simulink model "Pose_integration_R_L"  (R2016b)
settings: Solver=FixedStepDiscrete  StartTime=0.0  StopTime=60  FixedStep=0.02  RelTol=1e-3  EnableMultiTasking=on
InitFcn:
  | load('Pose_integration_R_L.mat')
StopFcn:
  | I = imread('Enviroment.png');
  | x = [0 35.9];
  | y=[23.31 0];
  | image(I,'XData',x,'YData',y);
  | axis xy;
  | hold on
  | plot (X.Data, Y.Data,'b');
  | plot (X1.Data, Y1.Data,'r');
undefined symbols (not defined in the file or in its folder): DiscIntNeverNeededParam, Ts
settings Model: Creator=antonio  LastModifiedBy=Antonio
settings DataIOCC: LimitDataPoints=on  SaveFormat=Array
settings OptimizationCC: LifeSpan=inf
settings DebuggingCC: UnderspecifiedInitializationDetection=Classic  MergeDetectMultiDrivingBlocksExec=none  SolverPrmCheckMsg=warning  StateNameClashWarn=warning  SFUnexpectedBacktrackingDiag=warning  SFNoUnconditionalDefaultTransitionDiag=warning  SFExecutionAtInitializationDiag=none
settings HardwareCC: ProdBitPerPointer=32  ProdBitPerSizeT=32  ProdBitPerPtrDiffT=32  ProdLargestAtomicFloat=None  ProdIntDivRoundTo=Undefined  ProdEndianess=Unspecified  ProdWordSize=32  ProdHWDeviceType=32-bit Generic
settings ModelReferenceCC: PropagateSignalLabelsOutOfModel=off
settings GRTTargetCC: TargetLangStandard=C89/C90 (ANSI)  GeneratePreprocessorConditionals=Disable all
settings ConfigComp: CovMetricSettings=dw  CovHtmlReporting=on  CovSaveCumulativeToWorkspaceVar=on  CovSaveSingleToWorkspaceVar=on  CovExternalEMLEnable=off

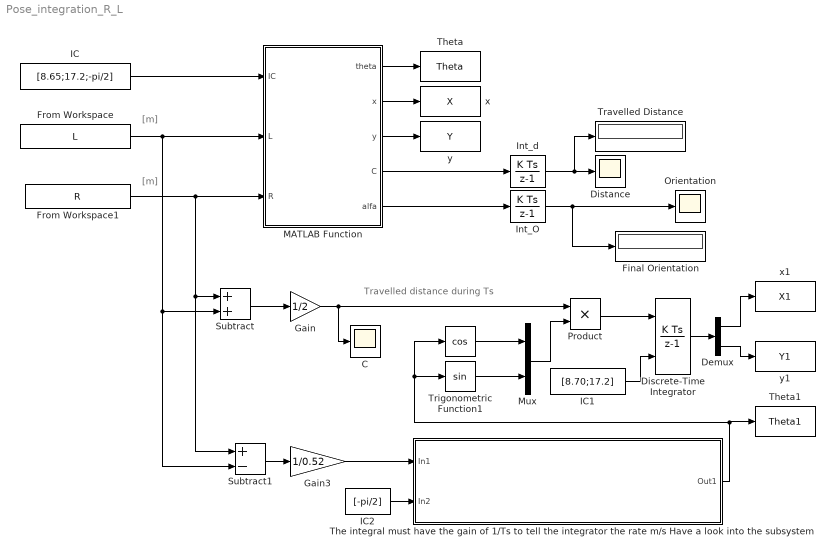
== system Pose_integration_R_L ==
  note: Travelled distance during Ts
  note: [m]
  note: [m]
  " " : Trigonometry  Operator=cos
  C : Scope
  Demux : Demux  Outputs=2
  Discrete-Time Integrator : DiscreteIntegrator  gainval=1/Ts  InitialConditionSource=external  InitialConditionSetting=State (most efficient)  SampleTime=Ts  ICPrevOutput=DiscIntNeverNeededParam  ICPrevScaledInput=DiscIntNeverNeededParam
  Distance : Scope
  Final Orientation : Display
  From Workspace : FromWorkspace  VariableName=L  SampleTime=0
  From Workspace1 : FromWorkspace  VariableName=R  SampleTime=0
  Gain : Gain  Gain=1/2
  Gain3 : Gain  Gain=1/0.52
  IC : Constant  Value=[8.65;17.2;-pi/2]
  IC1 : Constant  Value=[8.70;17.2]
  IC2 : Constant  Value=[-pi/2]
  Int_O : DiscreteIntegrator  gainval=1/Ts  InitialCondition=-pi/2  InitialConditionSetting=State (most efficient)  SampleTime=Ts  ICPrevOutput=DiscIntNeverNeededParam  ICPrevScaledInput=DiscIntNeverNeededParam
  Int_d : DiscreteIntegrator  gainval=1/Ts  InitialConditionSetting=State (most efficient)  SampleTime=Ts  ICPrevOutput=DiscIntNeverNeededParam  ICPrevScaledInput=DiscIntNeverNeededParam
  MATLAB Function : MATLAB Function  TreatAsAtomicUnit=on
  Mux : Mux  Inputs=2
  Orientation : Scope
  Product : Product
  Subtract : Sum
  Subtract1 : Sum  Inputs=+-
  The integral must have the gain of 1/Ts to tell the integrator the rate m/s Have a look into the subsystem : Subsystem
      mask Display: image('Integral.jpg');
  Theta : ToWorkspace  VariableName=Theta  SaveFormat=Timeseries  SampleTime=-1
  Theta1 : ToWorkspace  VariableName=Theta1  SaveFormat=Timeseries  SampleTime=-1
  Travelled Distance : Display
  Trigonometric Function1 : Trigonometry
  x : ToWorkspace  VariableName=X  SaveFormat=Timeseries  SampleTime=-1
  x1 : ToWorkspace  VariableName=X1  SaveFormat=Timeseries  SampleTime=-1
  y : ToWorkspace  VariableName=Y  SaveFormat=Timeseries  SampleTime=-1
  y1 : ToWorkspace  VariableName=Y1  SaveFormat=Timeseries  SampleTime=-1
  wires:
  IC/1 -> MATLAB Function/1(IC)
  MATLAB Function/1(theta) -> Theta/1
  MATLAB Function/3(y) -> y/1
  MATLAB Function/2(x) -> x/1
  From Workspace1/1 -> Subtract1/1, Subtract/1, MATLAB Function/3(R)
  From Workspace/1 -> MATLAB Function/2(L), Subtract1/2, Subtract/2
  Subtract/1 -> Gain/1
  Gain/1 -> C/1, Product/1
  Trigonometric Function1/1 -> Mux/2
  " "/1 -> Mux/1
  Mux/1 -> Product/2
  Subtract1/1 -> Gain3/1
  Product/1 -> Discrete-Time Integrator/1
  IC1/1 -> Discrete-Time Integrator/2
  Discrete-Time Integrator/1 -> Demux/1
  Demux/1 -> x1/1
  Demux/2 -> y1/1
  MATLAB Function/4(C) -> Int_d/1
  Int_d/1 -> Travelled Distance/1, Distance/1
  Int_O/1 -> Orientation/1, Final Orientation/1
  MATLAB Function/5(alfa) -> Int_O/1
  The integral must have the gain of 1/Ts to tell the integrator the rate m/s Have a look into the subsystem/1(Out1) -> " "/1, Trigonometric Function1/1, Theta1/1
  Gain3/1 -> The integral must have the gain of 1/Ts to tell the integrator the rate m/s Have a look into the subsystem/1(In1)
  IC2/1 -> The integral must have the gain of 1/Ts to tell the integrator the rate m/s Have a look into the subsystem/2(In2)

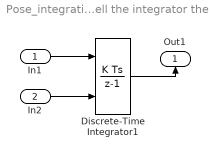
== system Pose_integration_R_L/The integral must have the gain of 1//Ts to tell the integrator the rate m//s Have a look into the subsystem ==
  In1 : Inport
  In2 : Inport  Port=2
  Discrete-Time Integrator1 : DiscreteIntegrator  gainval=1/Ts  InitialConditionSource=external  InitialConditionSetting=State (most efficient)  SampleTime=Ts  ICPrevOutput=DiscIntNeverNeededParam  ICPrevScaledInput=DiscIntNeverNeededParam
  Out1 : Outport
  wires:
  In1/1 -> Discrete-Time Integrator1/1
  In2/1 -> Discrete-Time Integrator1/2
  Discrete-Time Integrator1/1 -> Out1/1

== matlab function Pose_integration_R_L/MATLAB Function ==
  data: theta output; x output; IC input; y output; L input; R input; C output; alfa output
function [theta,x,y,C,alfa] = fcn(IC,L,R) % IC->Initial Condition [xo,yo,th0]
                                   % R and L are the displacements of
                                   % wheels [m]
persistent x_w y_w suma_theta %  internal variable to be mantain its values

ts=0.02; % sample time

%%%%%%%%%%%%%%%%%%%%%%%%%%%%%%%%%%%%%%%%%%%%%%%%%%%%%%%%%%%%%%%%%%%%%%%%%%
% %%%%%%%%%%%%%%   Read Initial condition   %%%%%%%%%%%%%%%%%%%%%%%%%%%%%%
x_ini=IC(1);
y_ini=IC(2);
theta_ini=IC(3);
%%%%%%%%%%%%%%%%%%%%%%%%%%%%%%%%%%%%%%%%%%%%%%%%%%%%%%%%%%%%%%%%%%%%%%%%%%
%%%%%%%%%%%%%%%   variable initialitation  %%%%%%%%%%%%%%%%%%%%%%%%%%%%%%
if isempty (x_w)
    x_w=x_ini;
end
if isempty (y_w)
    y_w=y_ini;
end
if isempty (suma_theta)
    suma_theta=theta_ini;
end
%%%%%%%%%%%%%%%%%%%%%%%%%%%%%%%%%%%%%%%%%%%%%%%%%%%%%%%%%%%%%%%%%%%%%%%%%%
%%%%%%%%%%%%%%%%%  compute the odometry    %%%%%%%%%%%%%%%%%%%%%%%%%%%%%%%
delta_th=........;
delta_d=.........;
%%%%%%%%%%%%%%%%%%%%%%%%%%%%%%%%%%%%%%%%%%%%%%%%%%%%%%%%%%%%%%%%%%%%%%%%%%
%%%%%%%%%%%%%%%%%  integration of the robot pose %%%%%%%%%%%%%%%%%%%%%%%%%%
x_w=x_w + ...........
y_w=y_w + ...........
suma_theta=mod(suma_theta+.........,2*pi); 
%%%%%%%%%%%%%%%%%%%%%%%%%%%%%%%%%%%%%%%%%%%%%%%%%%%%%%%%%%%%%%%%%%%%%%%%%%
%%%%%%%%%%%%%%%%%  output variable %%%%%%%%%%%%%%%%%%%%%%%%%%%%%%%%%%%%%%%

x=x_w;
y=y_w;
theta=suma_theta

end
